simulink model "InductionCoockerStateFlow_HarnessPowerLed"  (R2023a)
settings: Solver=FixedStepDiscrete  StartTime=0.0  StopTime=20  FixedStep=0.1  RelTol=1e-3  EnableMultiTasking=on
settings Model: Creator=antonio  LastModifiedBy=anton
settings SolverCC: AlgebraicLoopSolver=TrustRegion  AutoInsertRateTranBlk=on
settings DataIOCC: LimitDataPoints=on
settings OptimizationCC: LifeSpan=inf
settings DebuggingCC: UnconnectedInputMsg=warning  UnconnectedOutputMsg=warning  UnconnectedLineMsg=warning  AllowSymbolicDim=off  SFUnexpectedBacktrackingDiag=warning  SFNoUnconditionalDefaultTransitionDiag=warning  SFExecutionAtInitializationDiag=none  ArithmeticOperatorsInVariantConditions=warning
settings ModelReferenceCC: EnableRefExpFcnMdlSchedulingChecks=on
settings SFSimCC: SimUseLocalCustomCode=off  CustomCodeUndefinedFunction=UseInterfaceOnly
settings RTWCC: RTWUseLocalCustomCode=off  DLArmComputeVersion=19.05
settings CodeAppCC: StateflowObjectComments=on
settings GRTTargetCC: TargetLangStandard=C89/C90 (ANSI)
settings ConfigComp: CovEnable=on  RecordCoverage=on  CovMetricSettings=dw  CovSaveCumulativeToWorkspaceVar=on  CovSaveSingleToWorkspaceVar=on  CovModelRefEnable=on

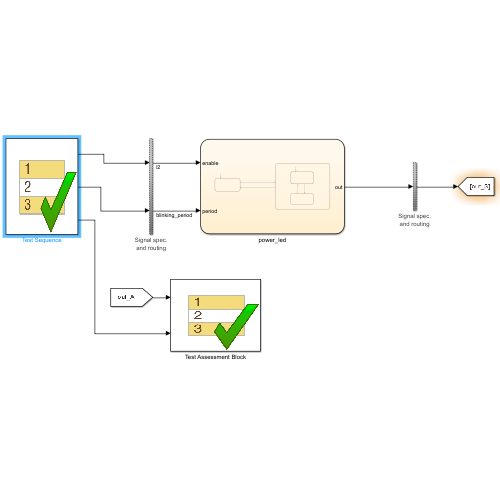
[thumbnail: Simulink's stored preview of the top-level diagram]
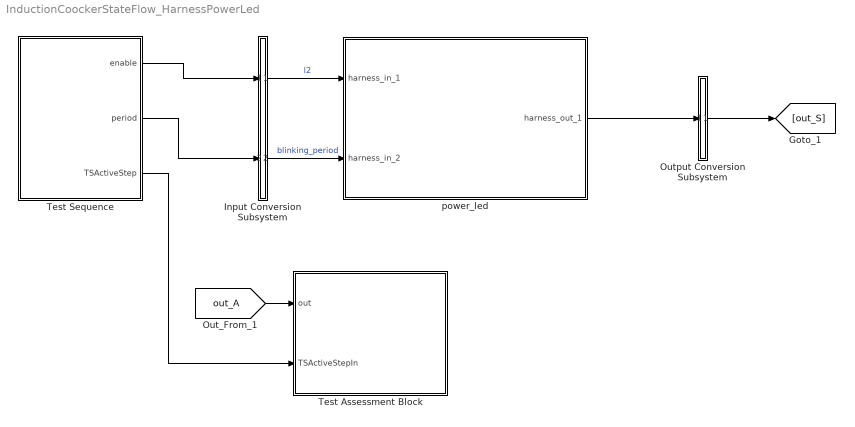
== system InductionCoockerStateFlow_HarnessPowerLed ==
  Input Conversion Subsystem : Subsystem  Tag=__SLT_ICS__  Description=|
      | Signal spec.
      | and routing
      settings: AttributesFormatString=%<Description>
  Output Conversion Subsystem : Subsystem  Tag=__SLT_OCS__  Description=|
      | Signal spec.
      | and routing
      settings: AttributesFormatString=%<Description>
  Test Assessment Block : Test Sequence  Tag=__SLT_ASMT__  TreatAsAtomicUnit=on
  Test Sequence : Test Sequence  TreatAsAtomicUnit=on
  power_led : Subsystem  Tag=__SL_testing_harness_stub_
  wires:
  [out_A] -> Test Assessment Block/1(out)
  Test Sequence/1(enable) -> Input Conversion Subsystem/1(Inport_1)
  Test Sequence/2(period) -> Input Conversion Subsystem/2(Inport_2)
  Output Conversion Subsystem/1(Outport_1) -> [out_S]
  Test Sequence/3(TSActiveStep) -> Test Assessment Block/2(TSActiveStepIn)
  power_led/1(harness_out_1) -> Output Conversion Subsystem/1(Inport_1)
  Input Conversion Subsystem/1(Outport_1) -> power_led/1(harness_in_1)  "l2"
  Input Conversion Subsystem/2(Outport_2) -> power_led/2(harness_in_2)  "blinking_period"

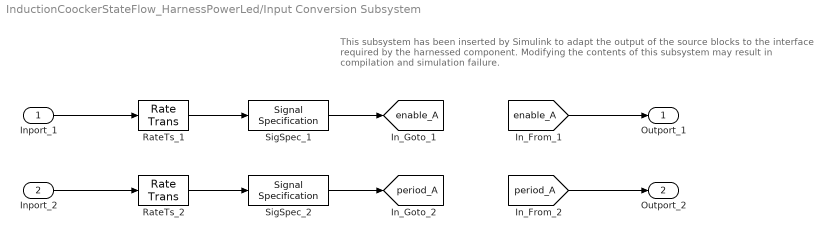
== system InductionCoockerStateFlow_HarnessPowerLed/Input Conversion Subsystem ==
  note: This subsystem has been inserted by Simulink to adapt the output of the source blocks to the interface required by the harnessed component.
      |  Modifying the contents of this subsystem may result in compilation and simulation failure.
  Inport_1 : Inport
  Inport_2 : Inport  Port=2
  RateTs_1 : RateTransition  OutPortSampleTime=0.1
  RateTs_2 : RateTransition  OutPortSampleTime=0.1
  SigSpec_1 : SignalSpecification  OutDataTypeStr=boolean  Dimensions=[1]  SampleTime=0.1
  SigSpec_2 : SignalSpecification  OutDataTypeStr=uint32  Dimensions=[1]  SampleTime=0.1
  Outport_1 : Outport
  Outport_2 : Outport  Port=2
  tag scope: enable_A=global, period_A=global
  wires:
  [enable_A] -> Outport_1/1
  SigSpec_1/1 -> [enable_A]
  RateTs_1/1 -> SigSpec_1/1
  Inport_1/1 -> RateTs_1/1
  [period_A] -> Outport_2/1
  SigSpec_2/1 -> [period_A]
  RateTs_2/1 -> SigSpec_2/1
  Inport_2/1 -> RateTs_2/1

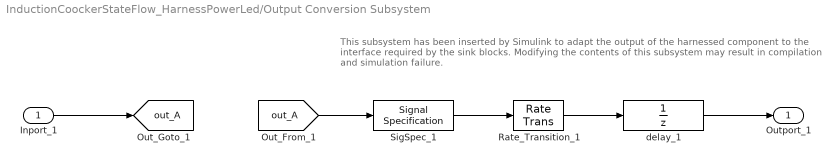
== system InductionCoockerStateFlow_HarnessPowerLed/Output Conversion Subsystem ==
  note: This subsystem has been inserted by Simulink to adapt the output of the harnessed component to the interface required by the sink blocks.
      |  Modifying the contents of this subsystem may result in compilation and simulation failure.
  Inport_1 : Inport
  Rate_Transition_1 : RateTransition  OutPortSampleTimeOpt=Inherit
  SigSpec_1 : SignalSpecification  OutDataTypeStr=boolean  Dimensions=[1]  SampleTime=0.1
  delay_1 : UnitDelay  SampleTime=-1
  Outport_1 : Outport
  tag scope: out_A=global
  wires:
  Inport_1/1 -> [out_A]
  [out_A] -> SigSpec_1/1
  SigSpec_1/1 -> Rate_Transition_1/1
  Rate_Transition_1/1 -> delay_1/1
  delay_1/1 -> Outport_1/1

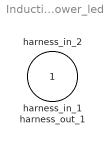
== system InductionCoockerStateFlow_HarnessPowerLed/power_led ==
  harness_in_1 : Inport
  harness_in_2 : Inport  Port=2
  harness_out_1 : Outport

== stateflow chart InductionCoockerStateFlow_HarnessPowerLed/Test Assessment Block ==
  state Scenario_1
    state Run
      state VerifyInit
        verify(~out)
      state VerifyLedIsEnabledOn
        verify(out)
      state VerifyLedIsEnabledOff
        verify(~out)
      state VerifyLedIsEnabledOnAgain
        verify(out)
      state VerifyLedIsNotEnabled
        verify(~out)
      state step_1_2
      (default) -> (junction 107)
      Run -> (junction 107)
      (junction 107) -> (junction 108) [order 1] : [TSActiveStepIn == TSActiveStepEnumPowerLed.Init
          | ]
      (junction 108) -> VerifyInit [order 1] : [~in(Scenario_1.Run.VerifyInit)]
      (junction 107) -> (junction 116) [order 2]
      (junction 108) -> (junction 111) [order 2]
      (junction 116) -> (junction 117) [order 1] : [TSActiveStepIn == TSActiveStepEnumPowerLed.LedIsEnabledOn
          | ]
      (junction 117) -> VerifyLedIsEnabledOn [order 1] : [~in(Scenario_1.Run.VerifyLedIsEnabledOn)]
      (junction 116) -> (junction 124) [order 2]
      (junction 117) -> (junction 120) [order 2]
      (junction 124) -> (junction 125) [order 1] : [TSActiveStepIn == TSActiveStepEnumPowerLed.LedIsEnabledOff
          | ]
      (junction 125) -> VerifyLedIsEnabledOff [order 1] : [~in(Scenario_1.Run.VerifyLedIsEnabledOff)]
      (junction 124) -> (junction 132) [order 2]
      (junction 125) -> (junction 128) [order 2]
      (junction 132) -> (junction 133) [order 1] : [TSActiveStepIn == TSActiveStepEnumPowerLed.LedIsEnabledOnAgain
          | ]
      (junction 133) -> VerifyLedIsEnabledOnAgain [order 1] : [~in(Scenario_1.Run.VerifyLedIsEnabledOnAgain)]
      (junction 132) -> (junction 141) [order 2]
      (junction 133) -> (junction 136) [order 2]
      (junction 141) -> (junction 142) [order 1] : [TSActiveStepIn == TSActiveStepEnumPowerLed.LedIsNotEnabled
          | ]
      (junction 142) -> VerifyLedIsNotEnabled [order 1] : [~in(Scenario_1.Run.VerifyLedIsNotEnabled)]
      (junction 141) -> (junction 166) [order 2]
      (junction 142) -> (junction 145) [order 2]
      (junction 166) -> (junction 167)
      (junction 167) -> step_1_2 [order 1] : [~in(Scenario_1.Run.step_1_2)]
      (junction 167) -> (junction 170) [order 2]
    (default) -> Run
  (default) -> Scenario_1 : {assert(Active_Scenario_Index == 1,'The value of Scenario Parameter ''Active_Scenario_Index'' is not valid. Use the index of the scenario to specify it.')}
  data: out input boolean size=[1]; TSActiveStepIn input; Active_Scenario_Index parameter =1

== stateflow chart InductionCoockerStateFlow_HarnessPowerLed/Test Sequence ==
  settings: updateMethod=DISCRETE  sampleTime=0.1
  state Scenario_1
    state Init
      %% Initialize data outputs.
      enable = false;
      period = 0;
      settings: description=Il led è inizialmente spento.
    state LedIsEnabledOn
      enable = true;
      period = 1000;
      settings: description=|
          | Il led viene abilitato e viene impostato un
          | periodo di blink pari a 1000 msec.
    state LedIsEnabledOff
      enable = true;
      period = 1000;
      settings: description=|
          | Il led resta abilitato con lo stesso periodo
          | blink.
    state LedIsEnabledOnAgain
      enable = true;
      period = 1000;
      settings: description=|
          | Il led resta abilitato con lo stesso periodo
          | blink.
    state LedIsNotEnabled
      enable = false;
      period = 0;
    (default) -> Init
    Init -> LedIsEnabledOn : [
        | true
        | ]
    LedIsEnabledOn -> LedIsEnabledOff : [
        | after(period, msec)
        | ]
    LedIsEnabledOff -> LedIsEnabledOnAgain : [
        | after(period, msec)
        | ]
    LedIsEnabledOnAgain -> LedIsNotEnabled : [
        | true
        | ]
  (default) -> Scenario_1 : {assert(Active_Scenario_Index == 1,'The value of Scenario Parameter ''Active_Scenario_Index'' is not valid. Use the index of the scenario to specify it.')}
  data: enable output boolean size=[1]; period output uint32 size=[1]; TSActiveStep output Enum: TSActiveStepEnumPowerLed; Active_Scenario_Index parameter =1
